simulink model "Motor_and_Nav_Model"  (R2025a)
settings: Solver=FixedStepAuto  StartTime=0.0  StopTime=20  FixedStep=0.0001  RelTol=1e-3
model workspace (MAT data in the model file):
  Brush_Damp = 1
  Cylin_height = 1
  Cylin_rad = 0.5
  Kb = 1
  Kt = 1
  L = 5
  La = 1
  Ml = 10
  Mr = 20
  N = 1
  Ra = 1
  TLoad = 0
  d = 0
  r = 0.05
libraries: simulink x1
settings Model: Creator=seana  LastModifiedBy=andor

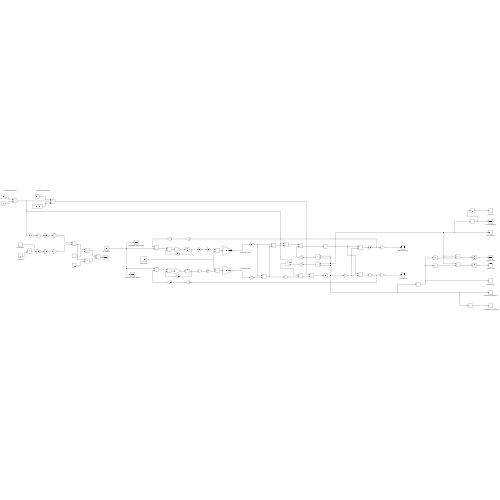
[thumbnail: Simulink's stored preview of the top-level diagram]
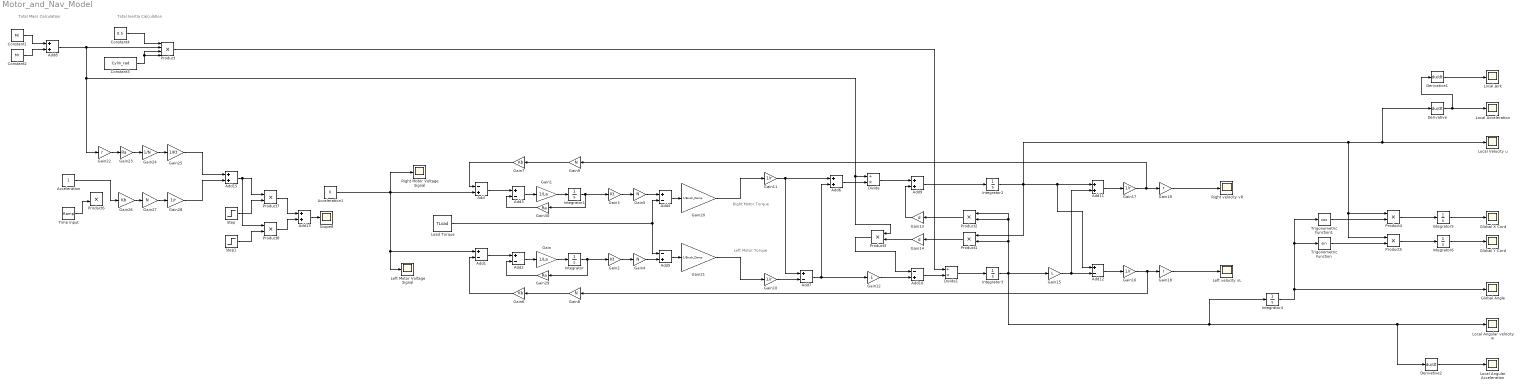
== system Motor_and_Nav_Model ==
  note: Left Motor Torque
  note: Right Motor Torque
  note: Total Mass Calculation
  note: Total Inertia Calculation
  Acceleration : Constant
  Acceleration1 : Constant  Value=0
  Add : Sum  Inputs=-+
  Add{1..4,7,12} (6 alike) : Sum  Inputs=+-
  Add10 : Sum  Inputs=-+
  Add{6,8..9,11,13,15} (6 alike) : Sum
  Add5 : Sum  Inputs=-+
  Constant1 : Constant  Value=Ml
  Constant2 : Constant  Value=Mr
  Constant3 : Constant  Value=Cylin_rad
  Constant4 : Constant  Value=0.5
  Derivative : Derivative
  Derivative1 : Derivative
  Derivative2 : Derivative
  Divide : Product  Inputs=/*
  Divide1 : Product  Inputs=/*
  Gain : Gain  Gain=1/La
  Gain1 : Gain  Gain=1/La
  Gain{10..11,16..17,28} (5 alike) : Gain  Gain=1/r
  Gain12 : Gain  Gain=L
  Gain13 : Gain  Gain=d
  Gain14 : Gain  Gain=d
  Gain15 : Gain  Gain=L
  Gain18 : Gain  Gain=r
  Gain19 : Gain  Gain=r
  Gain2 : Gain  Gain=Kt
  Gain20 : Gain  Gain=1/Brush_Damp
  Gain21 : Gain  Gain=1/Brush_Damp
  Gain22 : Gain  Gain=r
  Gain23 : Gain  Gain=Ra
  Gain24 : Gain  Gain=1/N
  Gain25 : Gain  Gain=1/Kt
  Gain26 : Gain  Gain=Kb
  Gain{4..5,8..9,27} (5 alike) : Gain  Gain=N
  Gain29 : Gain  Gain=Ra
  Gain3 : Gain  Gain=Kt
  Gain30 : Gain  Gain=Ra
  Gain6 : Gain  Gain=Kb
  Gain7 : Gain  Gain=Kb
  Global Angle : Scope
      settings: ActiveDisplayYMinimum=-1  ActiveDisplayYMaximum=1  DataLoggingVariableName=ScopeData6
  Global X Cord : Scope
      settings: ActiveDisplayYMinimum=-0.44728900532907423  ActiveDisplayYMaximum=0.94531282024862562  DataLoggingVariableName=ScopeData4
  Global Y Cord : Scope
      settings: ActiveDisplayYMinimum=-1.3443648153536685  ActiveDisplayYMaximum=1.3358264658963324  DataLoggingVariableName=ScopeData5
  Integrator{,1..6} (7 alike) : Integrator
  Left Motor Voltage Signal : Scope
      settings: ActiveDisplayYMinimum=-1.5825063929052026  ActiveDisplayYMaximum=15.131968469934135  DataLoggingVariableName=ScopeData7
  Left velocity vL : Scope
      settings: ActiveDisplayYMinimum=-1  ActiveDisplayYMaximum=1  DataLoggingVariableName=ScopeData3
  Load Torque : Constant  Value=TLoad
  Local Acceleration : Scope
      settings: ActiveDisplayYMinimum=-3.10199059707557  ActiveDisplayYMaximum=2.4934496486311142
  Local Angular Acceleration : Scope
      settings: ActiveDisplayYMinimum=-1  ActiveDisplayYMaximum=1  DataLoggingVariableName=ScopeData3
  Local Angular velocity w : Scope
      settings: ActiveDisplayYMinimum=-1  ActiveDisplayYMaximum=1
  Local Jerk : Scope
      settings: ActiveDisplayYMinimum=-0.5294  ActiveDisplayYMaximum=0.68792  DataLoggingVariableName=ScopeData2
  Local Velocity u : Scope
      settings: ActiveDisplayYMinimum=-0.966595141275304  ActiveDisplayYMaximum=2.7014437428215521
  Product : Product  Inputs=4
  Product{1..8} (8 alike) : Product
  Right Motor Voltage Signal : Scope
      settings: ActiveDisplayYMinimum=-0.53233967104510094  ActiveDisplayYMaximum=2.1193725740357943  DataLoggingVariableName=ScopeData9
  Right velocity vR : Scope
      settings: ActiveDisplayYMinimum=-1  ActiveDisplayYMaximum=1  DataLoggingVariableName=ScopeData2
  Scope8 : Scope
      settings: ActiveDisplayYMinimum=19.990630838402289  ActiveDisplayYMaximum=22.353711940173735  DataLoggingVariableName=ScopeData4
  Step : Step  Time=0  SampleTime=0
  Step1 : Step  After=-1  SampleTime=0
  Time Input : simulink/Sources/Ramp  slope=1  start=0  InitialOutput=0
  Trigonometric Function : Trigonometry
  Trigonometric Function1 : Trigonometry  Operator=cos
  wires:
  Add2/1 -> Gain/1
  Gain/1 -> Integrator/1
  Integrator/1 -> Gain29/1, Gain2/1
  Add3/1 -> Gain1/1
  Integrator1/1 -> Gain30/1, Gain3/1
  Gain1/1 -> Integrator1/1
  Add/1 -> Add3/1
  Add1/1 -> Add2/1
  Gain3/1 -> Gain5/1
  Gain2/1 -> Gain4/1
  Gain6/1 -> Add1/2
  Gain7/1 -> Add/1
  Gain9/1 -> Gain7/1
  Gain4/1 -> Add5/2
  Gain5/1 -> Add4/1
  Load Torque/1 -> Add4/2, Add5/1
  Gain10/1 -> Add7/2
  Gain11/1 -> Add7/1, Add6/1
  Add7/1 -> Gain12/1, Add6/2
  Constant1/1 -> Add8/1
  Constant2/1 -> Add8/2
  Constant3/1 -> Product/4, Product/3
  Add8/1 -> Gain22/1, Product3/1, Divide/1, Product/2
  Constant4/1 -> Product/1
  Add6/1 -> Divide/2
  Gain12/1 -> Add10/2
  Divide/1 -> Add9/1
  Product2/1 -> Gain13/1
  Gain13/1 -> Add9/2
  Product1/1 -> Gain14/1
  Gain14/1 -> Product3/2
  Product3/1 -> Add10/1
  Add9/1 -> Integrator2/1
  Add10/1 -> Divide1/2
  Divide1/1 -> Integrator3/1
  Product/1 -> Divide1/1
  Integrator3/1 -> Gain15/1, Integrator4/1, Derivative2/1, Local Angular velocity w/1, Product1/2, Product2/2, Product2/1
  Integrator2/1 -> Add12/1, Add11/1, Product1/1, Product4/1, Product5/1, Derivative/1, Local Velocity u/1
  Gain15/1 -> Add12/2, Add11/2
  Add11/1 -> Gain17/1
  Add12/1 -> Gain16/1
  Gain19/1 -> Right velocity vR/1
  Gain18/1 -> Left velocity vL/1
  Integrator4/1 -> Trigonometric Function/1, Trigonometric Function1/1, Global Angle/1
  Trigonometric Function1/1 -> Product4/2
  Trigonometric Function/1 -> Product5/2
  Product4/1 -> Integrator5/1
  Product5/1 -> Integrator6/1
  Integrator5/1 -> Global X Cord/1
  Integrator6/1 -> Global Y Cord/1
  Gain16/1 -> Gain8/1, Gain18/1
  Gain17/1 -> Gain9/1, Gain19/1
  Add4/1 -> Gain20/1
  Add5/1 -> Gain21/1
  Gain21/1 -> Gain10/1
  Gain20/1 -> Gain11/1
  Derivative/1 -> Local Acceleration/1, Derivative1/1
  Derivative1/1 -> Local Jerk/1
  Derivative2/1 -> Local Angular Acceleration/1
  Gain22/1 -> Gain23/1
  Gain23/1 -> Gain24/1
  Gain24/1 -> Gain25/1
  Gain26/1 -> Gain27/1
  Gain27/1 -> Gain28/1
  Gain28/1 -> Add15/2
  Gain25/1 -> Add15/1
  Time Input/1 -> Product6/2
  Step1/1 -> Product8/2
  Step/1 -> Product7/2
  Add15/1 -> Product8/1, Product7/1
  Product8/1 -> Add13/2
  Product7/1 -> Add13/1
  Acceleration1/1 -> Left Motor Voltage Signal/1, Add1/1, Add/2, Right Motor Voltage Signal/1
  Add13/1 -> Scope8/1
  Gain8/1 -> Gain6/1
  Gain29/1 -> Add2/2
  Gain30/1 -> Add3/2
  Acceleration/1 -> Gain26/1
